simulink model "LedSwitching"  (R2021b)
settings: Solver=FixedStepDiscrete  StartTime=0.0  StopTime=10.0  RelTol=1e-3  EnableMultiTasking=on
settings Model: Creator=fady  LastModifiedBy=fady
settings DataIOCC: ReturnWorkspaceOutputs=off
settings OptimizationCC: DefaultParameterBehavior=Inlined  InlineInvariantSignals=on  EnableMemcpy=off  LifeSpan=1  EfficientTunableParamExpr=on
settings DebuggingCC: UnderspecifiedInitializationDetection=Classic  MergeDetectMultiDrivingBlocksExec=none  SFMachineParentedDataDiag=warning  ArithmeticOperatorsInVariantConditions=warning
settings ModelReferenceCC: PropagateSignalLabelsOutOfModel=off
settings SFSimCC: MATLABDynamicMemAlloc=off  CustomCodeUndefinedFunction=UseInterfaceOnly
settings RTWCC: Description=Embedded Coder  SystemTargetFile=ert.tlc  GenCodeOnly=on  TemplateMakefile=ert_default_tmf  GenerateReport=on  IncludeHyperlinkInReport=on  LaunchReport=on  GenerateTraceInfo=on  GenerateTraceReport=on  GenerateTraceReportSl=on  GenerateTraceReportSf=on  GenerateTraceReportEml=on
settings CodeAppCC: ForceParamTrailComments=on  IgnoreCustomStorageClasses=off  OperatorAnnotations=on  SimulinkDataObjDesc=on  SFDataObjDesc=on  MATLABFcnDesc=on  InsertBlockDesc=on  StateflowObjectComments=on  MATLABSourceComments=on
settings ERTTargetCC: MultiwordLength=2048  GenerateSampleERTMain=on  InlinedParameterPlacement=NonHierarchical  ERTCustomFileTemplate=example_file_process.tlc

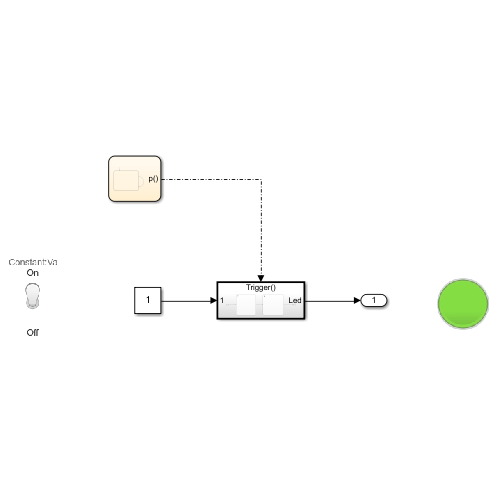
[thumbnail: Simulink's stored preview of the top-level diagram]
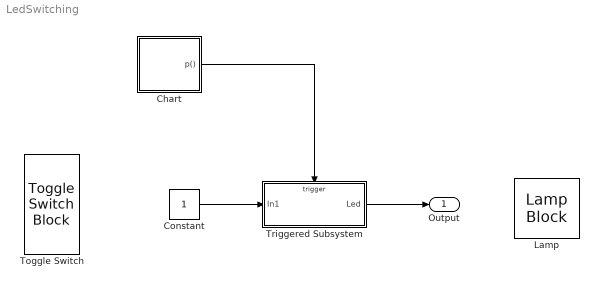
== system LedSwitching ==
  Chart : Stateflow chart  TreatAsAtomicUnit=on
  Constant : Constant
  Lamp : LampBlock  LabelPosition=Hide
  Toggle Switch : ToggleSwitchBlock
      settings: Values={{'Off', 'On'}, [0 1]}
  Triggered Subsystem : Subsystem  TreatAsAtomicUnit=on
  Output : Outport
  wires:
  Constant/1 -> Triggered Subsystem/1(In1)
  Triggered Subsystem/1(Led) -> Output/1
  Chart/1(p()) -> Triggered Subsystem/Trigger

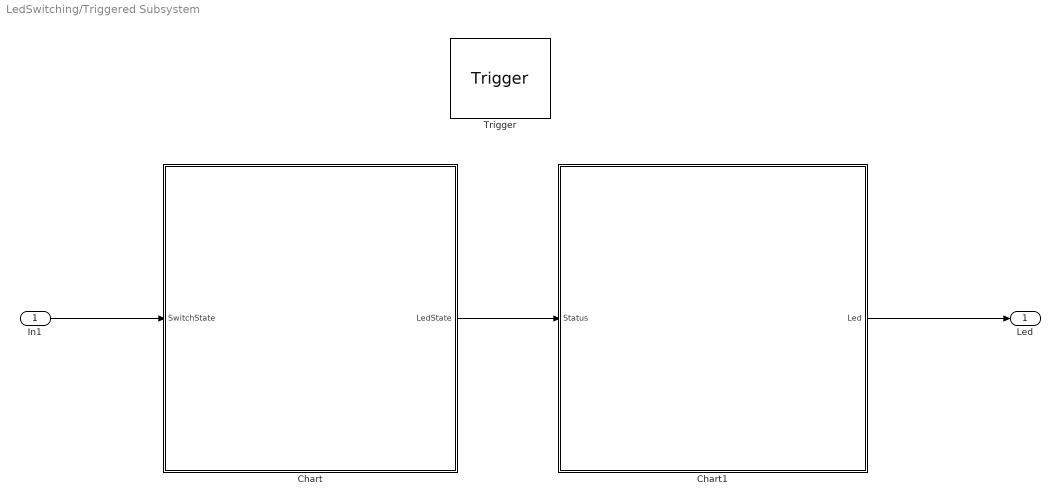
== system LedSwitching/Triggered Subsystem ==
  In1 : Inport
  Trigger : TriggerPort  TriggerType=function-call  VariantControl=(inherit)
  Chart : Stateflow chart  TreatAsAtomicUnit=on
  Chart1 : Stateflow chart  TreatAsAtomicUnit=on
  Led : Outport
  wires:
  In1/1 -> Chart/1(SwitchState)
  Chart/1(LedState) -> Chart1/1(Status)
  Chart1/1(Led) -> Led/1

== stateflow chart LedSwitching/Triggered Subsystem/Chart1 ==
  (default) -> (junction 7) : % Led_State
  (junction 7) -> (junction 8) [order 1] : [Status == 1]
  (junction 7) -> (junction 9) [order 2] : {Led  = 0;}
  (junction 8) -> (junction 10) : {Led = 1;}
  (junction 10) -> (junction 9)
  (junction 9) -> (junction 11)
  data: Status input; Led output

== stateflow chart LedSwitching/Chart ==
  state Counter
    en:
    ex:
  (default) -> Counter
  Counter -> Counter : [after(5,tick)]{p;}
  events: p output FUNCTION_CALL_EVENT

== stateflow chart LedSwitching/Triggered Subsystem/Chart ==
  (default) -> (junction 7) : % Switch_State
  (junction 7) -> (junction 8) [order 1] : [SwitchState == 1]
  (junction 7) -> (junction 9) [order 2] : {LedState = 0;}
  (junction 8) -> (junction 10) : {LedState = 1;}
  (junction 10) -> (junction 9)
  (junction 9) -> (junction 11)
  data: SwitchState input; LedState output
